simulink model "punto3"  (R2020b)
settings: Solver=VariableStepAuto  StartTime=0.0  StopTime=200  RelTol=1e-3
settings Model: Creator=User  LastModifiedBy=User

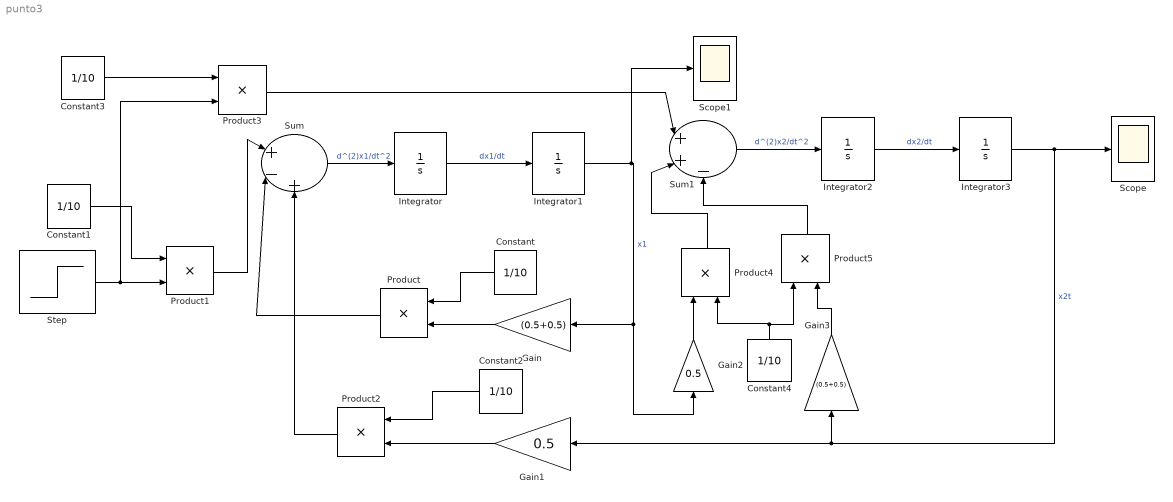
== system punto3 ==
  Constant{,1..4} (5 alike) : Constant  Value=1/10
  Gain : Gain  Gain=(0.5+0.5)
  Gain1 : Gain  Gain=0.5
  Gain2 : Gain  Gain=0.5
  Gain3 : Gain  Gain=(0.5+0.5)
  Integrator{,1..3} (4 alike) : Integrator
  Product{,1..5} (6 alike) : Product
  Scope : Scope
  Scope1 : Scope
  Step : Step  SampleTime=0
  Sum : Sum  Inputs=|+-+
  Sum1 : Sum  Inputs=|++-
  wires:
  Sum/1 -> Integrator/1  "d^(2)x1/dt^2"
  Integrator/1 -> Integrator1/1  "dx1/dt"
  Integrator1/1 -> Scope1/1, Gain/1, Gain2/1  "x1"
  Gain/1 -> Product/2
  Constant/1 -> Product/1
  Product/1 -> Sum/2
  Step/1 -> Product3/2, Product1/2
  Product1/1 -> Sum/1
  Constant1/1 -> Product1/1
  Sum1/1 -> Integrator2/1  "d^(2)x2/dt^2"
  Integrator2/1 -> Integrator3/1  "dx2/dt"
  Integrator3/1 -> Scope/1, Gain3/1, Gain1/1  "x2t"
  Gain1/1 -> Product2/2
  Constant2/1 -> Product2/1
  Product2/1 -> Sum/3
  Constant3/1 -> Product3/1
  Product3/1 -> Sum1/1
  Gain2/1 -> Product4/1
  Constant4/1 -> Product5/1, Product4/2
  Product4/1 -> Sum1/2
  Product5/1 -> Sum1/3
  Gain3/1 -> Product5/2
